simulink model "control_block_diagram copy"  (R2025b)
settings: Solver=VariableStepAuto  StartTime=0.0  StopTime=10.0  RelTol=1e-3
PreLoadFcn:
  | load 'Control Block Diagram'\contact_force.mat
model workspace (MAT data in the model file):
  B_imp = 1
  INA125_gain = 604
  J_imp = 1
  K_d = 1
  K_f = 1
  K_i = 1
  K_imp = 1
  K_p = 1
  finger_length = 0.105
  full_ROM = 90
  joint_pulley_diam = 0.1
  motor_pulley_diam = 0
  sine_freq_Hz = 2
  total_encoder_counts = 4096
undefined symbols (not defined in the file or in its folder): DiscIntNeverNeededParam
libraries: simulink x3
settings Model: Creator=Madeline  LastModifiedBy=Madeline

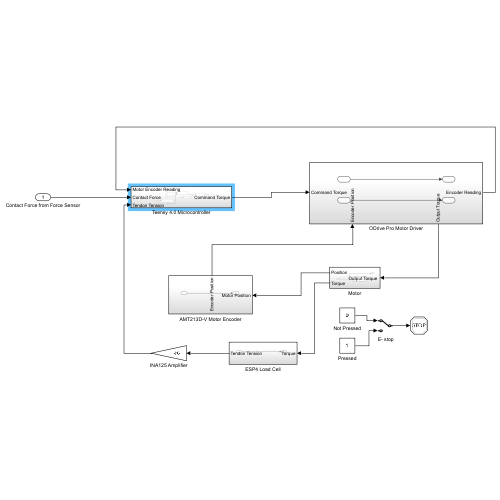
[thumbnail: Simulink's stored preview of the top-level diagram]
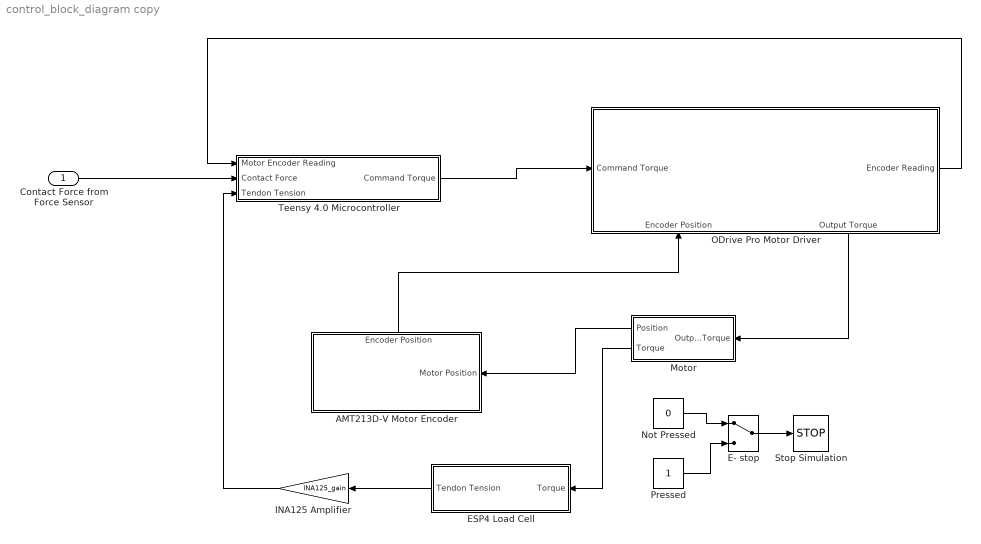
== system control_block_diagram copy ==
  Contact Force from Force Sensor : Inport
  " E- stop" : ManualSwitch
  AMT213D-V Motor Encoder : Subsystem
      settings: PortSchema="{\"entries\":[{\"content\":{\"sides\":[{\"content\":{\"connectorIds\":[\"In1\"]},\"type\":\"ConnectorPlacement.EquallySpacedRectSide\",\"uuid\":\"88afd67f-3209-48d2-80be-27a9c6027e98\"},{\"content\":{\"side\":\"RIGHT\"},\"type\":\"ConnectorPlacement.EquallySpacedRectSide\",\"uuid\":\"6bd83a64-80e2-4e6b-a2e1-60e2a1b1e7d1\"},{\"content\":{\"connectorIds\":[\"Out1\"],\"side\":\"TOP\"},\"type\":\"ConnectorPlacement.EquallySpacedRectSide\",\"uuid\":\"ca5e5761-7c4c-4ffd-94f8-cf864c9b5854\"}]},\"type\":\"ConnectorPlacement.EquallySpacedConnector\",\"uuid\":\"578619f2-0797-4ece-88f8-3f0e3f24fe58\"}],\"packageUris\":[\"http://schema.mathworks.com/mf0/Connector/R2020b\"],\"version\":\"1.0\"}"
  ESP4 Load Cell : Subsystem
  INA125 Amplifier : Gain  Gain=INA125_gain
  Motor : Subsystem
  Not Pressed : Constant  Value=0
  ODrive Pro Motor Driver : Subsystem
      settings: PortSchema="{\"entries\":[{\"content\":{\"sides\":[{\"content\":{\"connectorIds\":[\"In1\"]},\"type\":\"ConnectorPlacement.EquallySpacedRectSide\",\"uuid\":\"c97f3b25-cb08-4b77-804d-5691f1a52caa\"},{\"content\":{\"connectorIds\":[\"Out1\"],\"side\":\"RIGHT\"},\"type\":\"ConnectorPlacement.EquallySpacedRectSide\",\"uuid\":\"fc8ddf87-a458-4f73-a642-c7dd3d8cebff\"},{\"content\":{\"side\":\"TOP\"},\"type\":\"ConnectorPlacement.EquallySpacedRectSide\",\"uuid\":\"bec86457-f3cb-49fd-a085-c16f63c32d9e\"},{\"content\":{\"connectorIds\":[\"In2\",\"Out2\"],\"side\":\"BOTTOM\"},\"type\":\"ConnectorPlacement.EquallySpacedRectSide\",\"uuid\":\"4c0a5cbf-4f1d-4d43-a541-d1307432e3c9\"}]},\"type\":\"ConnectorPlacement.EquallySpacedConnector\",\"uuid\":\"94b3d347-19f8-405c-b5ff-c5a65504f3eb\"}],\"packageUris\":[\"http://schema.mathworks.com/mf0/Connector/R2020b\"],\"version\":\"1.0\"}"
  Pressed : Constant
  Stop Simulation : Stop
  Teensy 4.0 Microcontroller : Subsystem
  wires:
  ODrive Pro Motor Driver/2("Output Torque ") -> Motor/1("Output Torque ")
  Motor/1("Position ") -> AMT213D-V Motor Encoder/1(Motor Position)
  Teensy 4.0 Microcontroller/1(Command Torque) -> ODrive Pro Motor Driver/1(Command Torque)
  Contact Force from Force Sensor/1 -> Teensy 4.0 Microcontroller/2(Contact Force)
  AMT213D-V Motor Encoder/1(Encoder Position) -> ODrive Pro Motor Driver/2(Encoder Position)
  ODrive Pro Motor Driver/1(Encoder Reading) -> Teensy 4.0 Microcontroller/1(Motor Encoder Reading)
  Motor/2(Torque) -> ESP4 Load Cell/1(Torque)
  Not Pressed/1 -> " E- stop"/1
  Pressed/1 -> " E- stop"/2
  " E- stop"/1 -> Stop Simulation/1
  ESP4 Load Cell/1(Tendon Tension) -> INA125 Amplifier/1
  INA125 Amplifier/1 -> Teensy 4.0 Microcontroller/3(Tendon Tension)

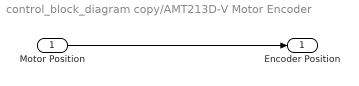
== system control_block_diagram copy/AMT213D-V Motor Encoder ==
  Motor Position : Inport
  Encoder Position : Outport
  wires:
  Motor Position/1 -> Encoder Position/1

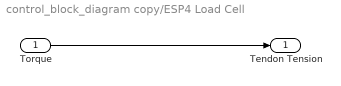
== system control_block_diagram copy/ESP4 Load Cell ==
  Torque : Inport
  Tendon Tension : Outport
  wires:
  Torque/1 -> Tendon Tension/1

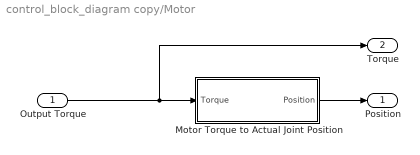
== system control_block_diagram copy/Motor ==
  "Output Torque " : Inport
  Motor Torque to Actual Joint Position : Subsystem
  "Position " : Outport
  Torque : Outport  Port=2
  wires:
  Motor Torque to Actual Joint Position/1(Position) -> "Position "/1
  "Output Torque "/1 -> Motor Torque to Actual Joint Position/1("Torque "), Torque/1

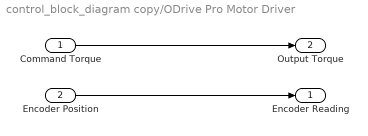
== system control_block_diagram copy/ODrive Pro Motor Driver ==
  Command Torque : Inport
  Encoder Position : Inport  Port=2
  Encoder Reading : Outport
  "Output Torque " : Outport  Port=2
  wires:
  Command Torque/1 -> "Output Torque "/1
  Encoder Position/1 -> Encoder Reading/1

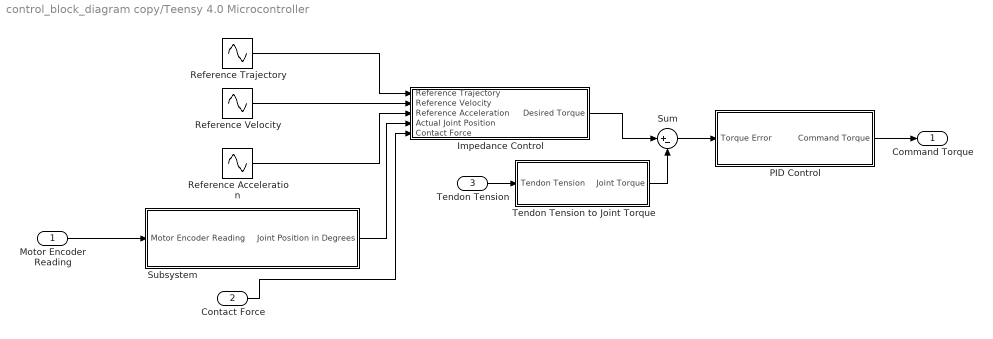
== system control_block_diagram copy/Teensy 4.0 Microcontroller ==
  Motor Encoder Reading : Inport
  Contact Force : Inport  Port=2
  Tendon Tension : Inport  Port=3
  Impedance Control : Subsystem
  PID Control : Subsystem
  Reference Acceleration : Sin  Amplitude=-0.75*full_ROM*(sine_freq_Hz*2*pi)^2  Frequency=sine_freq_Hz*2*pi  SampleTime=0
  Reference Trajectory : Sin  Amplitude=0.75*full_ROM  Frequency=sine_freq_Hz*2*pi  SampleTime=0
  Reference Velocity : Sin  Amplitude=0.75*full_ROM*sine_freq_Hz*2*pi  Frequency=sine_freq_Hz*2*pi  Phase=pi/2  SampleTime=0
  Subsystem : Subsystem
  Sum : Sum  Inputs=|+-
  Tendon Tension to Joint Torque : Subsystem
  Command Torque : Outport
  wires:
  Sum/1 -> PID Control/1(Torque Error)
  PID Control/1(Command Torque) -> Command Torque/1
  Motor Encoder Reading/1 -> Subsystem/1(Motor Encoder Reading)
  Reference Trajectory/1 -> Impedance Control/1(Reference Trajectory)
  Contact Force/1 -> Impedance Control/5(Contact Force)
  Subsystem/1(Joint Position in Degrees) -> Impedance Control/4(Actual Joint Position)
  Reference Velocity/1 -> Impedance Control/2(Reference Velocity)
  Reference Acceleration/1 -> Impedance Control/3(Reference Acceleration)
  Impedance Control/1(Desired Torque) -> Sum/1
  Tendon Tension/1 -> Tendon Tension to Joint Torque/1(Tendon Tension)
  Tendon Tension to Joint Torque/1(Joint Torque) -> Sum/2

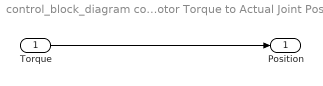
== system control_block_diagram copy/Motor/Motor Torque to Actual Joint Position ==
  "Torque " : Inport
  Position : Outport
  wires:
  "Torque "/1 -> Position/1

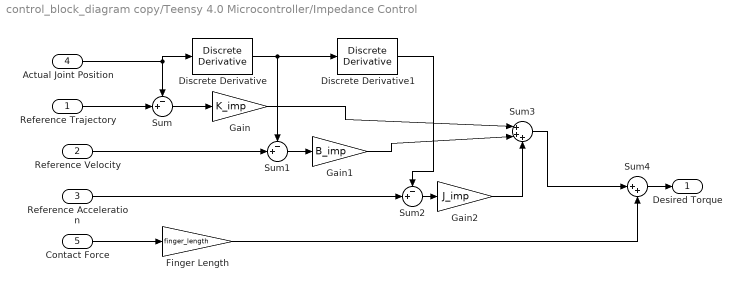
== system control_block_diagram copy/Teensy 4.0 Microcontroller/Impedance Control ==
  Reference Trajectory : Inport
  Reference Velocity : Inport  Port=2
  Reference Acceleration : Inport  Port=3
  Actual Joint Position : Inport  Port=4
  Contact Force : Inport  Port=5
  Discrete Derivative : simulink/Discrete/Discrete Derivative  gainval=1.0  ICPrevScaledInput=0.0  OutMin=[]  OutMax=[]  OutDataType=fixdt(1, 16)  OutScaling=2^-10  DoSatur=off
  Discrete Derivative1 : simulink/Discrete/Discrete Derivative  gainval=1.0  ICPrevScaledInput=0.0  OutMin=[]  OutMax=[]  OutDataType=fixdt(1, 16)  OutScaling=2^-10  DoSatur=off
  Finger Length : Gain  Gain=finger_length
  Gain : Gain  Gain=K_imp
  Gain1 : Gain  Gain=B_imp
  Gain2 : Gain  Gain=J_imp
  Sum : Sum  Inputs=-+|
  Sum1 : Sum  Inputs=-+|
  Sum2 : Sum  Inputs=-+|
  Sum3 : Sum  Inputs=|+++
  Sum4 : Sum  Inputs=|++
  Desired Torque : Outport
  wires:
  Reference Trajectory/1 -> Sum/2
  Actual Joint Position/1 -> Sum/1, Discrete Derivative/1
  Discrete Derivative/1 -> Sum1/1, Discrete Derivative1/1
  Reference Velocity/1 -> Sum1/2
  Discrete Derivative1/1 -> Sum2/1
  Reference Acceleration/1 -> Sum2/2
  Sum/1 -> Gain/1
  Sum1/1 -> Gain1/1
  Sum2/1 -> Gain2/1
  Gain/1 -> Sum3/1
  Gain1/1 -> Sum3/2
  Gain2/1 -> Sum3/3
  Contact Force/1 -> Finger Length/1
  Finger Length/1 -> Sum4/2
  Sum3/1 -> Sum4/1
  Sum4/1 -> Desired Torque/1

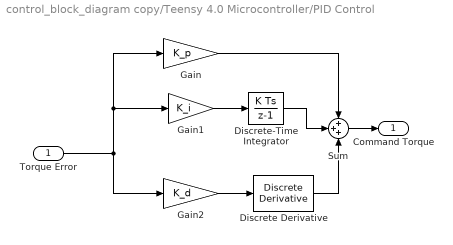
== system control_block_diagram copy/Teensy 4.0 Microcontroller/PID Control ==
  Torque Error : Inport
  Discrete Derivative : simulink/Discrete/Discrete Derivative  gainval=1.0  ICPrevScaledInput=0.0  OutMin=[]  OutMax=[]  OutDataType=fixdt(1, 16)  OutScaling=2^-10  DoSatur=off
  Discrete-Time Integrator : DiscreteIntegrator  SampleTime=-1  ICPrevOutput=DiscIntNeverNeededParam  ICPrevScaledInput=DiscIntNeverNeededParam
  Gain : Gain  Gain=K_p
  Gain1 : Gain  Gain=K_i
  Gain2 : Gain  Gain=K_d
  Sum : Sum  Inputs=+++
  Command Torque : Outport
  wires:
  Torque Error/1 -> Gain2/1, Gain/1, Gain1/1
  Gain2/1 -> Discrete Derivative/1
  Gain1/1 -> Discrete-Time Integrator/1
  Gain/1 -> Sum/1
  Discrete-Time Integrator/1 -> Sum/2
  Discrete Derivative/1 -> Sum/3
  Sum/1 -> Command Torque/1

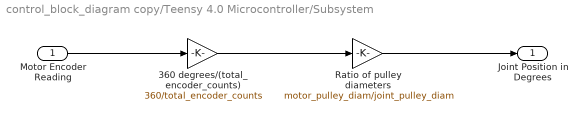
== system control_block_diagram copy/Teensy 4.0 Microcontroller/Subsystem ==
  Motor Encoder Reading : Inport
  360 degrees/(total_encoder_counts) : Gain  Gain=360/total_encoder_counts
  Ratio of pulley diameters : Gain  Gain=motor_pulley_diam/joint_pulley_diam
  Joint Position in Degrees : Outport
  wires:
  Motor Encoder Reading/1 -> 360 degrees/(total_encoder_counts)/1
  360 degrees/(total_encoder_counts)/1 -> Ratio of pulley diameters/1
  Ratio of pulley diameters/1 -> Joint Position in Degrees/1

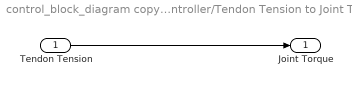
== system control_block_diagram copy/Teensy 4.0 Microcontroller/Tendon Tension to Joint Torque ==
  Tendon Tension : Inport
  Joint Torque : Outport
  wires:
  Tendon Tension/1 -> Joint Torque/1
